simulink model "SlidingMode"  (R2018a)
settings: Solver=FixedStepAuto  StartTime=0.0  StopTime=10.0  MaxStep=1e-2  RelTol=1e-5
PreLoadFcn:
  | modelDir = fileparts(get_param(bdroot, 'FileName'));
  | addpath(fullfile(modelDir,'../../Parameters'));
  | addpath(fullfile(modelDir,'../../Controllers/SlidingMode'));
  | 
  | Constants_Kugle
  | Constants_nominal
  | 
  | Parameters_Controllers
InitFcn:
  | Constants_Kugle
  | Constants_nominal
  | 
  | Parameters_Controllers
values from neighbouring files (symbols this model uses):
  K = [50.2853305369 -25.1426652685 -25.1426652685 6.08906467254e-15 43.5483736827 -43.5483736827 -4.08248290464 -4.08248290464 -4.08248290464 7.38986278673 -3.69493139337 -3.69493139337 ... (18 elements, 3x6)]    [LQRgains.mat]
undefined symbols (not defined in the file or in its folder): COM_nominal, constants_nominal, epsilon, eta, max_output_torque, SaturationTorqueOfMaxOutputTorque, SlidingManifold, SwitchingLaw
settings Model: Creator=thomas  LastModifiedBy=Thomas

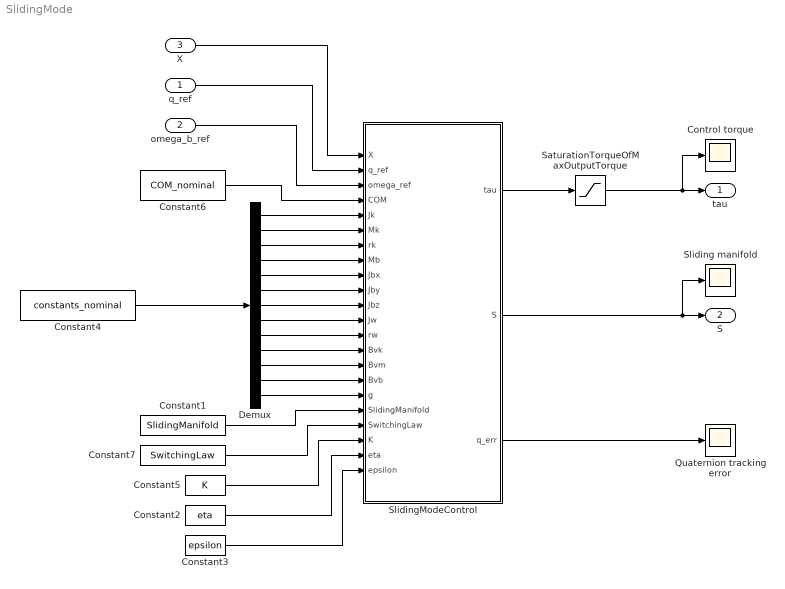
== system SlidingMode ==
  q_ref : Inport  PortDimensions=4
  omega_b_ref : Inport  Port=2  PortDimensions=3
  X : Inport  Port=3  PortDimensions=12
  Constant1 : Constant  Value=SlidingManifold
  Constant2 : Constant  Value=eta
  Constant3 : Constant  Value=epsilon
  Constant4 : Constant  Value=constants_nominal
  Constant5 : Constant  Value=K
  Constant6 : Constant  Value=COM_nominal
  Constant7 : Constant  Value=SwitchingLaw
  Control torque : Scope
  Demux : Demux  Outputs=13
  Quaternion tracking error : Scope
  SaturationTorqueOfMaxOutputTorque : Saturate  UpperLimit=SaturationTorqueOfMaxOutputTorque*max_output_torque  LowerLimit=-SaturationTorqueOfMaxOutputTorque*max_output_torque
  Sliding manifold : Scope
  SlidingModeControl : MATLAB Function  TreatAsAtomicUnit=on
  tau : Outport
  S : Outport  Port=2
  wires:
  Constant4/1 -> Demux/1
  Constant5/1 -> SlidingModeControl/20(K)
  SlidingModeControl/1(tau) -> SaturationTorqueOfMaxOutputTorque/1
  SlidingModeControl/3(q_err) -> Quaternion tracking error/1
  Demux/1 -> SlidingModeControl/5(Jk)
  Demux/2 -> SlidingModeControl/6(Mk)
  Demux/3 -> SlidingModeControl/7(rk)
  Demux/4 -> SlidingModeControl/8(Mb)
  Demux/5 -> SlidingModeControl/9(Jbx)
  Demux/6 -> SlidingModeControl/10(Jby)
  Demux/7 -> SlidingModeControl/11(Jbz)
  Demux/8 -> SlidingModeControl/12(Jw)
  Demux/9 -> SlidingModeControl/13(rw)
  Demux/10 -> SlidingModeControl/14(Bvk)
  Demux/11 -> SlidingModeControl/15(Bvm)
  Demux/13 -> SlidingModeControl/17(g)
  Demux/12 -> SlidingModeControl/16(Bvb)
  Constant6/1 -> SlidingModeControl/4(COM)
  X/1 -> SlidingModeControl/1(X)
  q_ref/1 -> SlidingModeControl/2(q_ref)
  omega_b_ref/1 -> SlidingModeControl/3(omega_ref)
  SlidingModeControl/2(S) -> Sliding manifold/1, S/1
  Constant1/1 -> SlidingModeControl/18(SlidingManifold)
  Constant2/1 -> SlidingModeControl/21(eta)
  Constant3/1 -> SlidingModeControl/22(epsilon)
  Constant7/1 -> SlidingModeControl/19(SwitchingLaw)
  SaturationTorqueOfMaxOutputTorque/1 -> tau/1, Control torque/1

== matlab function SlidingMode/SlidingModeControl ==
  data: X input size=12; q_ref input size=4; omega_ref input size=3; COM input size=3; Jk input; Mk input; rk input; Mb input; Jbx input; Jby input; Jbz input; Jw input; rw input; Bvk input; Bvm input; Bvb input; g input; SlidingManifold input; SwitchingLaw input; K input; tau output size=3; S output; q_err output size=4; eta input; epsilon input
function [tau, S, q_err] = SlidingModeControl_(X,q_ref,omega_ref,  COM,Jk,Mk,rk,Mb,Jbx,Jby,Jbz,Jw,rw,Bvk,Bvm,Bvb,g,  SlidingManifold,SwitchingLaw,K,eta,epsilon)
    COM_X = COM(1);
    COM_Y = COM(2);
    COM_Z = COM(3);
    
    [tau, S, q_err] = SlidingModeControl(X,q_ref,omega_ref,  COM_X,COM_Y,COM_Z,Jbx,Jby,Jbz,Jk,Jw,Mb,Mk,Bvb,Bvk,Bvm,rk,rw,g,  SlidingManifold,SwitchingLaw,K,eta,epsilon);
end
